simulink model "gap_generation_single_veh"  (R2019a)
settings: Solver=VariableStepAuto  StartTime=0.0  StopTime=35  FixedStep=0.1  MaxStep=0.05  RelTol=1e-3
libraries: simulink x21, powerlib_meascontrol x5, autolibshared x5
(part 2 of 3)

== system gap_generation_single_veh/Fo/Longitudinal Adjustments for Lane Change ==
  currentStates : Inport
  leaderStates : Inport  Port=2
  lcFlag : Inport  Port=3
  Enable : EnablePort
  Bus Selector : BusSelector  OutputSignals=X,Xdot,u
  Bus Selector1 : BusSelector  OutputSignals=X,Xdot
  Chart : Stateflow chart  BlockKeywords=__PRM__SERIALIZED__DATA__:Stateflow Chart,Stateflow Diagram  TreatAsAtomicUnit=on
  Gain3 : Gain  Gain=velFilterGain/10
  Headway error : Subsystem
  Input Saturation : Saturate  UpperLimit=maxComfAccel  LowerLimit=minComfAccel
  Integrator1 : Integrator  InitialCondition=vx0
  Mux : Mux  Inputs=2
  Rate Limiter : RateLimiter  RisingSlewLimit=maxComfJerk  FallingSlewLimit=minComfJerk  SampleTimeMode=inherited
  Saturation : Saturate  UpperLimit=maxAcceleration  LowerLimit=minAcceleration
  Scope3 : Scope  NumInputPorts=2
  Sum : Sum  Inputs=-+|
  Sum2 : Sum  Inputs=|+-
  Sum6 : Sum  Inputs=|+-
  Transport Delay : TransportDelay  DelayTime=0.01
  Transport Delay1 : TransportDelay  DelayTime=0.01
  Veh Following : Subsystem  TreatAsAtomicUnit=on
  Velocity Control : Subsystem  TreatAsAtomicUnit=on
  vMin : Constant  Value=vMin
  u : Outport  InitialOutput=0
  errors : Outport  Port=2  OutputWhenDisabled=reset  InitialOutput=[0, 0]
  gap : Outport  Port=3  OutputWhenDisabled=reset  InitialOutput=[0]
  wires:
  Transport Delay1/1 -> Velocity Control/1(intReset)
  Chart/1(state) -> Transport Delay1/1
  Transport Delay/1 -> Scope3/1, Input Saturation/1
  Velocity Control/1(Out1) -> Chart/2(uVelControl)  "uVelControl"
  Veh Following/1(u) -> Chart/3(uVehFoll)  "uVehFoll"
  Saturation/1 -> Integrator1/1
  Input Saturation/1 -> Rate Limiter/1
  Rate Limiter/1 -> Scope3/2, u/1  "sat(u)"
  Headway error/1(eh) -> Veh Following/1(eh), Mux/1  "eh"
  Sum2/1 -> Gain3/1
  Sum6/1 -> Velocity Control/2(ev), Chart/1(velDiff)
  Bus Selector1/2 -> Sum2/1  "<Xdot>"
  Chart/2(u) -> Transport Delay/1  "u"
  Sum/1 -> Veh Following/2(ev), Mux/2  "ev"
  vMin/1 -> Sum6/1
  Gain3/1 -> Saturation/1
  Integrator1/1 -> Sum2/2, Sum/2
  Mux/1 -> errors/1
  Bus Selector/2 -> Sum6/2, Sum/1, Headway error/2(vf)  "<Xdot>"
  Bus Selector/1 -> Headway error/1(xf)  "<X>"
  currentStates/1 -> Bus Selector/1
  Headway error/2("gap ") -> gap/1
  leaderStates/1 -> Bus Selector1/1
  Bus Selector1/1 -> Headway error/3(xl)  "<X>"
  lcFlag/1 -> Headway error/4(lcFlag)
  Bus Selector/3 -> Veh Following/3(realInput)  "<u>"

== system gap_generation_single_veh/Fo/Regular Vehicle Following ==
  currentStates : Inport
  leaderStates : Inport  Port=2
  lcFlag : Inport  Port=3
  AND1 : Logic  IconShape=distinctive  AllPortsSameDT=off  OutDataTypeStr=boolean
  Bus Selector : BusSelector  OutputSignals=X,Xdot,u
  Bus Selector1 : BusSelector  OutputSignals=X,Xdot
  Compare To Constant : simulink/Logic and Bit Operations/Compare To Constant  relop=<  const=2*maxHeadwayError  OutDataTypeStr=boolean
  Gain3 : Gain  Gain=velFilterGain
  Headway error : Subsystem
  Integrator1 : Integrator  InitialCondition=vx0
  Merge : Merge
  Mux : Mux  Inputs=2
  NOT : Logic  Operator=NOT  IconShape=distinctive  AllPortsSameDT=off  OutDataTypeStr=boolean
  NOT1 : Logic  Operator=NOT  IconShape=distinctive  AllPortsSameDT=off  OutDataTypeStr=boolean
  Rate Limiter : RateLimiter  RisingSlewLimit=maxJerk  FallingSlewLimit=minJerk  SampleTimeMode=inherited
  Rate Limiter1 : RateLimiter  RisingSlewLimit=maxComfJerk  FallingSlewLimit=minComfJerk  SampleTimeMode=inherited
  Saturation : Saturate  UpperLimit=maxAcceleration  LowerLimit=minAcceleration
  Sum : Sum  Inputs=-+|
  Sum2 : Sum  Inputs=|+-
  Switch1 : Switch  Criteria=u2 > Threshold
  Transport Delay : TransportDelay  DelayTime=0.01
  Veh Following : Subsystem  TreatAsAtomicUnit=on
  Velocity Control : Subsystem  TreatAsAtomicUnit=on
  comf saturation : Saturate  UpperLimit=maxComfAccel  LowerLimit=minComfAccel
  safe saturation : Saturate  UpperLimit=maxAcceleration  LowerLimit=minAcceleration
  u : Outport
  errors : Outport  Port=2
  gap : Outport  Port=3
  wires:
  NOT1/1 -> Velocity Control/Enable
  lcFlag/1 -> Headway error/4(lcFlag), AND1/1
  NOT/1 -> AND1/2
  Bus Selector/3 -> Veh Following/3(realInput)  "<u>"
  Bus Selector1/1 -> Headway error/3(xl)  "<X>"
  Headway error/3(unsafeFlag) -> NOT/1
  Headway error/2("gap ") -> gap/1
  Headway error/1(eh) -> Compare To Constant/1, Veh Following/1(eh), Mux/1
  Mux/1 -> errors/1
  Transport Delay/1 -> comf saturation/1, safe saturation/1
  Merge/1 -> Transport Delay/1
  Velocity Control/1(Out1) -> Merge/2
  Compare To Constant/1 -> Veh Following/Enable, NOT1/1
  Veh Following/1(u) -> Merge/1
  Rate Limiter1/1 -> Switch1/1  "sat(u)"
  Switch1/1 -> u/1
  Rate Limiter/1 -> Switch1/3  "sat(u)"
  safe saturation/1 -> Rate Limiter/1
  AND1/1 -> Switch1/2
  comf saturation/1 -> Rate Limiter1/1
  leaderStates/1 -> Bus Selector1/1
  Bus Selector/1 -> Headway error/1(xf)  "<X>"
  currentStates/1 -> Bus Selector/1
  Sum/1 -> Velocity Control/1(ev), Veh Following/2(ev), Mux/2
  Sum2/1 -> Gain3/1
  Bus Selector1/2 -> Sum2/1  "<Xdot>"
  Integrator1/1 -> Sum/2, Sum2/2
  Saturation/1 -> Integrator1/1
  Gain3/1 -> Saturation/1
  Bus Selector/2 -> Headway error/2(vf), Sum/1  "<Xdot>"

== system gap_generation_single_veh/Ld/Longitudinal Adjustments for Lane Change ==
  currentStates : Inport
  leaderStates : Inport  Port=2
  lcFlag : Inport  Port=3
  Enable : EnablePort
  Bus Selector : BusSelector  OutputSignals=X,Xdot,u
  Bus Selector1 : BusSelector  OutputSignals=X,Xdot
  Chart : Stateflow chart  BlockKeywords=__PRM__SERIALIZED__DATA__:Stateflow Chart,Stateflow Diagram  TreatAsAtomicUnit=on
  Gain3 : Gain  Gain=velFilterGain/10
  Headway error : Subsystem
  Input Saturation : Saturate  UpperLimit=maxComfAccel  LowerLimit=minComfAccel
  Integrator1 : Integrator  InitialCondition=vx0
  Mux : Mux  Inputs=2
  Rate Limiter : RateLimiter  RisingSlewLimit=maxComfJerk  FallingSlewLimit=minComfJerk  SampleTimeMode=inherited
  Saturation : Saturate  UpperLimit=maxAcceleration  LowerLimit=minAcceleration
  Scope3 : Scope  NumInputPorts=2
  Sum : Sum  Inputs=-+|
  Sum2 : Sum  Inputs=|+-
  Sum6 : Sum  Inputs=|+-
  Transport Delay : TransportDelay  DelayTime=0.01
  Transport Delay1 : TransportDelay  DelayTime=0.01
  Veh Following : Subsystem  TreatAsAtomicUnit=on
  Velocity Control : Subsystem  TreatAsAtomicUnit=on
  vMin : Constant  Value=vMin
  u : Outport  InitialOutput=0
  errors : Outport  Port=2  OutputWhenDisabled=reset  InitialOutput=[0, 0]
  gap : Outport  Port=3  OutputWhenDisabled=reset  InitialOutput=[0]
  wires:
  Transport Delay1/1 -> Velocity Control/1(intReset)
  Chart/1(state) -> Transport Delay1/1
  Transport Delay/1 -> Scope3/1, Input Saturation/1
  Velocity Control/1(Out1) -> Chart/2(uVelControl)  "uVelControl"
  Veh Following/1(u) -> Chart/3(uVehFoll)  "uVehFoll"
  Saturation/1 -> Integrator1/1
  Input Saturation/1 -> Rate Limiter/1
  Rate Limiter/1 -> Scope3/2, u/1  "sat(u)"
  Headway error/1(eh) -> Veh Following/1(eh), Mux/1  "eh"
  Sum2/1 -> Gain3/1
  Sum6/1 -> Velocity Control/2(ev), Chart/1(velDiff)
  Bus Selector1/2 -> Sum2/1  "<Xdot>"
  Chart/2(u) -> Transport Delay/1  "u"
  Sum/1 -> Veh Following/2(ev), Mux/2  "ev"
  vMin/1 -> Sum6/1
  Gain3/1 -> Saturation/1
  Integrator1/1 -> Sum2/2, Sum/2
  Mux/1 -> errors/1
  Bus Selector/2 -> Sum6/2, Sum/1, Headway error/2(vf)  "<Xdot>"
  Bus Selector/1 -> Headway error/1(xf)  "<X>"
  currentStates/1 -> Bus Selector/1
  Headway error/2("gap ") -> gap/1
  leaderStates/1 -> Bus Selector1/1
  Bus Selector1/1 -> Headway error/3(xl)  "<X>"
  lcFlag/1 -> Headway error/4(lcFlag)
  Bus Selector/3 -> Veh Following/3(realInput)  "<u>"

== system gap_generation_single_veh/Ld/Regular Vehicle Following ==
  currentStates : Inport
  leaderStates : Inport  Port=2
  lcFlag : Inport  Port=3
  AND1 : Logic  IconShape=distinctive  AllPortsSameDT=off  OutDataTypeStr=boolean
  Bus Selector : BusSelector  OutputSignals=X,Xdot,u
  Bus Selector1 : BusSelector  OutputSignals=X,Xdot
  Compare To Constant : simulink/Logic and Bit Operations/Compare To Constant  relop=<  const=2*maxHeadwayError  OutDataTypeStr=boolean
  Gain3 : Gain  Gain=velFilterGain
  Headway error : Subsystem
  Integrator1 : Integrator  InitialCondition=vx0
  Merge : Merge
  Mux : Mux  Inputs=2
  NOT : Logic  Operator=NOT  IconShape=distinctive  AllPortsSameDT=off  OutDataTypeStr=boolean
  NOT1 : Logic  Operator=NOT  IconShape=distinctive  AllPortsSameDT=off  OutDataTypeStr=boolean
  Rate Limiter : RateLimiter  RisingSlewLimit=maxJerk  FallingSlewLimit=minJerk  SampleTimeMode=inherited
  Rate Limiter1 : RateLimiter  RisingSlewLimit=maxComfJerk  FallingSlewLimit=minComfJerk  SampleTimeMode=inherited
  Saturation : Saturate  UpperLimit=maxAcceleration  LowerLimit=minAcceleration
  Sum : Sum  Inputs=-+|
  Sum2 : Sum  Inputs=|+-
  Switch1 : Switch  Criteria=u2 > Threshold
  Transport Delay : TransportDelay  DelayTime=0.01
  Veh Following : Subsystem  TreatAsAtomicUnit=on
  Velocity Control : Subsystem  TreatAsAtomicUnit=on
  comf saturation : Saturate  UpperLimit=maxComfAccel  LowerLimit=minComfAccel
  safe saturation : Saturate  UpperLimit=maxAcceleration  LowerLimit=minAcceleration
  u : Outport
  errors : Outport  Port=2
  gap : Outport  Port=3
  wires:
  NOT1/1 -> Velocity Control/Enable
  lcFlag/1 -> Headway error/4(lcFlag), AND1/1
  NOT/1 -> AND1/2
  Bus Selector/3 -> Veh Following/3(realInput)  "<u>"
  Bus Selector1/1 -> Headway error/3(xl)  "<X>"
  Headway error/3(unsafeFlag) -> NOT/1
  Headway error/2("gap ") -> gap/1
  Headway error/1(eh) -> Compare To Constant/1, Veh Following/1(eh), Mux/1
  Mux/1 -> errors/1
  Transport Delay/1 -> comf saturation/1, safe saturation/1
  Merge/1 -> Transport Delay/1
  Velocity Control/1(Out1) -> Merge/2
  Compare To Constant/1 -> Veh Following/Enable, NOT1/1
  Veh Following/1(u) -> Merge/1
  Rate Limiter1/1 -> Switch1/1  "sat(u)"
  Switch1/1 -> u/1
  Rate Limiter/1 -> Switch1/3  "sat(u)"
  safe saturation/1 -> Rate Limiter/1
  AND1/1 -> Switch1/2
  comf saturation/1 -> Rate Limiter1/1
  leaderStates/1 -> Bus Selector1/1
  Bus Selector/1 -> Headway error/1(xf)  "<X>"
  currentStates/1 -> Bus Selector/1
  Sum/1 -> Velocity Control/1(ev), Veh Following/2(ev), Mux/2
  Sum2/1 -> Gain3/1
  Bus Selector1/2 -> Sum2/1  "<Xdot>"
  Integrator1/1 -> Sum/2, Sum2/2
  Saturation/1 -> Integrator1/1
  Gain3/1 -> Saturation/1
  Bus Selector/2 -> Headway error/2(vf), Sum/1  "<Xdot>"

== system gap_generation_single_veh/Lo/Longitudinal Adjustments for Lane Change ==
  currentStates : Inport
  leaderStates : Inport  Port=2
  lcFlag : Inport  Port=3
  Enable : EnablePort
  Bus Selector : BusSelector  OutputSignals=X,Xdot,u
  Bus Selector1 : BusSelector  OutputSignals=X,Xdot
  Chart : Stateflow chart  BlockKeywords=__PRM__SERIALIZED__DATA__:Stateflow Chart,Stateflow Diagram  TreatAsAtomicUnit=on
  Gain3 : Gain  Gain=velFilterGain/10
  Headway error : Subsystem
  Input Saturation : Saturate  UpperLimit=maxComfAccel  LowerLimit=minComfAccel
  Integrator1 : Integrator  InitialCondition=vx0
  Mux : Mux  Inputs=2
  Rate Limiter : RateLimiter  RisingSlewLimit=maxComfJerk  FallingSlewLimit=minComfJerk  SampleTimeMode=inherited
  Saturation : Saturate  UpperLimit=maxAcceleration  LowerLimit=minAcceleration
  Scope3 : Scope  NumInputPorts=2
  Sum : Sum  Inputs=-+|
  Sum2 : Sum  Inputs=|+-
  Sum6 : Sum  Inputs=|+-
  Transport Delay : TransportDelay  DelayTime=0.01
  Transport Delay1 : TransportDelay  DelayTime=0.01
  Veh Following : Subsystem  TreatAsAtomicUnit=on
  Velocity Control : Subsystem  TreatAsAtomicUnit=on
  vMin : Constant  Value=vMin
  u : Outport  InitialOutput=0
  errors : Outport  Port=2  OutputWhenDisabled=reset  InitialOutput=[0, 0]
  gap : Outport  Port=3  OutputWhenDisabled=reset  InitialOutput=[0]
  wires:
  Transport Delay1/1 -> Velocity Control/1(intReset)
  Chart/1(state) -> Transport Delay1/1
  Transport Delay/1 -> Scope3/1, Input Saturation/1
  Velocity Control/1(Out1) -> Chart/2(uVelControl)  "uVelControl"
  Veh Following/1(u) -> Chart/3(uVehFoll)  "uVehFoll"
  Saturation/1 -> Integrator1/1
  Input Saturation/1 -> Rate Limiter/1
  Rate Limiter/1 -> Scope3/2, u/1  "sat(u)"
  Headway error/1(eh) -> Veh Following/1(eh), Mux/1  "eh"
  Sum2/1 -> Gain3/1
  Sum6/1 -> Velocity Control/2(ev), Chart/1(velDiff)
  Bus Selector1/2 -> Sum2/1  "<Xdot>"
  Chart/2(u) -> Transport Delay/1  "u"
  Sum/1 -> Veh Following/2(ev), Mux/2  "ev"
  vMin/1 -> Sum6/1
  Gain3/1 -> Saturation/1
  Integrator1/1 -> Sum2/2, Sum/2
  Mux/1 -> errors/1
  Bus Selector/2 -> Sum6/2, Sum/1, Headway error/2(vf)  "<Xdot>"
  Bus Selector/1 -> Headway error/1(xf)  "<X>"
  currentStates/1 -> Bus Selector/1
  Headway error/2("gap ") -> gap/1
  leaderStates/1 -> Bus Selector1/1
  Bus Selector1/1 -> Headway error/3(xl)  "<X>"
  lcFlag/1 -> Headway error/4(lcFlag)
  Bus Selector/3 -> Veh Following/3(realInput)  "<u>"

== system gap_generation_single_veh/Lo/Regular Vehicle Following ==
  currentStates : Inport
  leaderStates : Inport  Port=2
  lcFlag : Inport  Port=3
  AND1 : Logic  IconShape=distinctive  AllPortsSameDT=off  OutDataTypeStr=boolean
  Bus Selector : BusSelector  OutputSignals=X,Xdot,u
  Bus Selector1 : BusSelector  OutputSignals=X,Xdot
  Compare To Constant : simulink/Logic and Bit Operations/Compare To Constant  relop=<  const=2*maxHeadwayError  OutDataTypeStr=boolean
  Gain3 : Gain  Gain=velFilterGain
  Headway error : Subsystem
  Integrator1 : Integrator  InitialCondition=vx0
  Merge : Merge
  Mux : Mux  Inputs=2
  NOT : Logic  Operator=NOT  IconShape=distinctive  AllPortsSameDT=off  OutDataTypeStr=boolean
  NOT1 : Logic  Operator=NOT  IconShape=distinctive  AllPortsSameDT=off  OutDataTypeStr=boolean
  Rate Limiter : RateLimiter  RisingSlewLimit=maxJerk  FallingSlewLimit=minJerk  SampleTimeMode=inherited
  Rate Limiter1 : RateLimiter  RisingSlewLimit=maxComfJerk  FallingSlewLimit=minComfJerk  SampleTimeMode=inherited
  Saturation : Saturate  UpperLimit=maxAcceleration  LowerLimit=minAcceleration
  Sum : Sum  Inputs=-+|
  Sum2 : Sum  Inputs=|+-
  Switch1 : Switch  Criteria=u2 > Threshold
  Transport Delay : TransportDelay  DelayTime=0.01
  Veh Following : Subsystem  TreatAsAtomicUnit=on
  Velocity Control : Subsystem  TreatAsAtomicUnit=on
  comf saturation : Saturate  UpperLimit=maxComfAccel  LowerLimit=minComfAccel
  safe saturation : Saturate  UpperLimit=maxAcceleration  LowerLimit=minAcceleration
  u : Outport
  errors : Outport  Port=2
  gap : Outport  Port=3
  wires:
  NOT1/1 -> Velocity Control/Enable
  lcFlag/1 -> Headway error/4(lcFlag), AND1/1
  NOT/1 -> AND1/2
  Bus Selector/3 -> Veh Following/3(realInput)  "<u>"
  Bus Selector1/1 -> Headway error/3(xl)  "<X>"
  Headway error/3(unsafeFlag) -> NOT/1
  Headway error/2("gap ") -> gap/1
  Headway error/1(eh) -> Compare To Constant/1, Veh Following/1(eh), Mux/1
  Mux/1 -> errors/1
  Transport Delay/1 -> comf saturation/1, safe saturation/1
  Merge/1 -> Transport Delay/1
  Velocity Control/1(Out1) -> Merge/2
  Compare To Constant/1 -> Veh Following/Enable, NOT1/1
  Veh Following/1(u) -> Merge/1
  Rate Limiter1/1 -> Switch1/1  "sat(u)"
  Switch1/1 -> u/1
  Rate Limiter/1 -> Switch1/3  "sat(u)"
  safe saturation/1 -> Rate Limiter/1
  AND1/1 -> Switch1/2
  comf saturation/1 -> Rate Limiter1/1
  leaderStates/1 -> Bus Selector1/1
  Bus Selector/1 -> Headway error/1(xf)  "<X>"
  currentStates/1 -> Bus Selector/1
  Sum/1 -> Velocity Control/1(ev), Veh Following/2(ev), Mux/2
  Sum2/1 -> Gain3/1
  Bus Selector1/2 -> Sum2/1  "<Xdot>"
  Integrator1/1 -> Sum/2, Sum2/2
  Saturation/1 -> Integrator1/1
  Gain3/1 -> Saturation/1
  Bus Selector/2 -> Headway error/2(vf), Sum/1  "<Xdot>"

== system gap_generation_single_veh/p1/Longitudinal Adjustments for Lane Change ==
  currentStates : Inport
  leaderStates : Inport  Port=2
  lcFlag : Inport  Port=3
  Enable : EnablePort
  Bus Selector : BusSelector  OutputSignals=X,Xdot,u
  Bus Selector1 : BusSelector  OutputSignals=X,Xdot
  Chart : Stateflow chart  BlockKeywords=__PRM__SERIALIZED__DATA__:Stateflow Chart,Stateflow Diagram  TreatAsAtomicUnit=on
  Gain3 : Gain  Gain=velFilterGain/10
  Headway error : Subsystem
  Input Saturation : Saturate  UpperLimit=maxComfAccel  LowerLimit=minComfAccel
  Integrator1 : Integrator  InitialCondition=vx0
  Mux : Mux  Inputs=2
  Rate Limiter : RateLimiter  RisingSlewLimit=maxComfJerk  FallingSlewLimit=minComfJerk  SampleTimeMode=inherited
  Saturation : Saturate  UpperLimit=maxAcceleration  LowerLimit=minAcceleration
  Scope3 : Scope  NumInputPorts=2
  Sum : Sum  Inputs=-+|
  Sum2 : Sum  Inputs=|+-
  Sum6 : Sum  Inputs=|+-
  Transport Delay : TransportDelay  DelayTime=0.01
  Transport Delay1 : TransportDelay  DelayTime=0.01
  Veh Following : Subsystem  TreatAsAtomicUnit=on
  Velocity Control : Subsystem  TreatAsAtomicUnit=on
  vMin : Constant  Value=vMin
  u : Outport  InitialOutput=0
  errors : Outport  Port=2  OutputWhenDisabled=reset  InitialOutput=[0, 0]
  gap : Outport  Port=3  OutputWhenDisabled=reset  InitialOutput=[0]
  wires:
  Transport Delay1/1 -> Velocity Control/1(intReset)
  Chart/1(state) -> Transport Delay1/1
  Transport Delay/1 -> Scope3/1, Input Saturation/1
  Velocity Control/1(Out1) -> Chart/2(uVelControl)  "uVelControl"
  Veh Following/1(u) -> Chart/3(uVehFoll)  "uVehFoll"
  Saturation/1 -> Integrator1/1
  Input Saturation/1 -> Rate Limiter/1
  Rate Limiter/1 -> Scope3/2, u/1  "sat(u)"
  Headway error/1(eh) -> Veh Following/1(eh), Mux/1  "eh"
  Sum2/1 -> Gain3/1
  Sum6/1 -> Velocity Control/2(ev), Chart/1(velDiff)
  Bus Selector1/2 -> Sum2/1  "<Xdot>"
  Chart/2(u) -> Transport Delay/1  "u"
  Sum/1 -> Veh Following/2(ev), Mux/2  "ev"
  vMin/1 -> Sum6/1
  Gain3/1 -> Saturation/1
  Integrator1/1 -> Sum2/2, Sum/2
  Mux/1 -> errors/1
  Bus Selector/2 -> Sum6/2, Sum/1, Headway error/2(vf)  "<Xdot>"
  Bus Selector/1 -> Headway error/1(xf)  "<X>"
  currentStates/1 -> Bus Selector/1
  Headway error/2("gap ") -> gap/1
  leaderStates/1 -> Bus Selector1/1
  Bus Selector1/1 -> Headway error/3(xl)  "<X>"
  lcFlag/1 -> Headway error/4(lcFlag)
  Bus Selector/3 -> Veh Following/3(realInput)  "<u>"

== system gap_generation_single_veh/p1/Regular Vehicle Following ==
  currentStates : Inport
  leaderStates : Inport  Port=2
  lcFlag : Inport  Port=3
  AND1 : Logic  IconShape=distinctive  AllPortsSameDT=off  OutDataTypeStr=boolean
  Bus Selector : BusSelector  OutputSignals=X,Xdot,u
  Bus Selector1 : BusSelector  OutputSignals=X,Xdot
  Compare To Constant : simulink/Logic and Bit Operations/Compare To Constant  relop=<  const=2*maxHeadwayError  OutDataTypeStr=boolean
  Gain3 : Gain  Gain=velFilterGain
  Headway error : Subsystem
  Integrator1 : Integrator  InitialCondition=vx0
  Merge : Merge
  Mux : Mux  Inputs=2
  NOT : Logic  Operator=NOT  IconShape=distinctive  AllPortsSameDT=off  OutDataTypeStr=boolean
  NOT1 : Logic  Operator=NOT  IconShape=distinctive  AllPortsSameDT=off  OutDataTypeStr=boolean
  Rate Limiter : RateLimiter  RisingSlewLimit=maxJerk  FallingSlewLimit=minJerk  SampleTimeMode=inherited
  Rate Limiter1 : RateLimiter  RisingSlewLimit=maxComfJerk  FallingSlewLimit=minComfJerk  SampleTimeMode=inherited
  Saturation : Saturate  UpperLimit=maxAcceleration  LowerLimit=minAcceleration
  Sum : Sum  Inputs=-+|
  Sum2 : Sum  Inputs=|+-
  Switch1 : Switch  Criteria=u2 > Threshold
  Transport Delay : TransportDelay  DelayTime=0.01
  Veh Following : Subsystem  TreatAsAtomicUnit=on
  Velocity Control : Subsystem  TreatAsAtomicUnit=on
  comf saturation : Saturate  UpperLimit=maxComfAccel  LowerLimit=minComfAccel
  safe saturation : Saturate  UpperLimit=maxAcceleration  LowerLimit=minAcceleration
  u : Outport
  errors : Outport  Port=2
  gap : Outport  Port=3
  wires:
  NOT1/1 -> Velocity Control/Enable
  lcFlag/1 -> Headway error/4(lcFlag), AND1/1
  NOT/1 -> AND1/2
  Bus Selector/3 -> Veh Following/3(realInput)  "<u>"
  Bus Selector1/1 -> Headway error/3(xl)  "<X>"
  Headway error/3(unsafeFlag) -> NOT/1
  Headway error/2("gap ") -> gap/1
  Headway error/1(eh) -> Compare To Constant/1, Veh Following/1(eh), Mux/1
  Mux/1 -> errors/1
  Transport Delay/1 -> comf saturation/1, safe saturation/1
  Merge/1 -> Transport Delay/1
  Velocity Control/1(Out1) -> Merge/2
  Compare To Constant/1 -> Veh Following/Enable, NOT1/1
  Veh Following/1(u) -> Merge/1
  Rate Limiter1/1 -> Switch1/1  "sat(u)"
  Switch1/1 -> u/1
  Rate Limiter/1 -> Switch1/3  "sat(u)"
  safe saturation/1 -> Rate Limiter/1
  AND1/1 -> Switch1/2
  comf saturation/1 -> Rate Limiter1/1
  leaderStates/1 -> Bus Selector1/1
  Bus Selector/1 -> Headway error/1(xf)  "<X>"
  currentStates/1 -> Bus Selector/1
  Sum/1 -> Velocity Control/1(ev), Veh Following/2(ev), Mux/2
  Sum2/1 -> Gain3/1
  Bus Selector1/2 -> Sum2/1  "<Xdot>"
  Integrator1/1 -> Sum/2, Sum2/2
  Saturation/1 -> Integrator1/1
  Gain3/1 -> Saturation/1
  Bus Selector/2 -> Headway error/2(vf), Sum/1  "<Xdot>"

== system gap_generation_single_veh/Fd/Longitudinal Adjustments for Lane Change/Headway error ==
  xf : Inport
  vf : Inport  Port=2
  xl : Inport  Port=3
  lcFlag : Inport  Port=4
  Demux : Demux  Outputs=2
  Integrator : Integrator  InitialCondition=h
  Multiply : Product
  Mux : Mux  Inputs=2
  Mux1 : Mux  Inputs=2
  Sum : Sum  Inputs=-+|
  Sum1 : Sum  Inputs=++|
  Sum2 : Sum  Inputs=+-|
  Sum3 : Sum  Inputs=|++
  Sum4 : Sum  Inputs=|+-
  Switch : Switch  Criteria=u2 > Threshold
  d0 : Constant  Value=d0
  d0Lc : Constant  Value=d0Lc
  h : Constant  Value=h
  hFilterGain : Gain  Gain=hFilterGain
  hLc : Constant  Value=hLc
  vLen : Constant  Value=lr+lf
  eh : Outport
  "gap " : Outport  Port=2
  wires:
  vLen/1 -> Sum1/1
  Multiply/1 -> Sum3/1
  Sum/1 -> "gap "/1, Sum2/1  "gap"
  xf/1 -> Sum1/2
  Sum3/1 -> Sum2/2  "desired  gap"
  vf/1 -> Multiply/1
  Sum1/1 -> Sum/1  "x (front bumber)"
  xl/1 -> Sum/2
  h/1 -> Mux/1
  Switch/1 -> Sum4/1
  hFilterGain/1 -> Integrator/1
  Sum4/1 -> hFilterGain/1
  Integrator/1 -> Sum4/2, Demux/1
  lcFlag/1 -> Switch/2
  Sum2/1 -> eh/1
  d0/1 -> Mux/2
  Mux/1 -> Switch/3
  hLc/1 -> Mux1/1
  d0Lc/1 -> Mux1/2
  Mux1/1 -> Switch/1
  Demux/1 -> Multiply/2  "time headway"
  Demux/2 -> Sum3/2  "gap at  standstill"

== system gap_generation_single_veh/Fd/Longitudinal Adjustments for Lane Change/Veh Following ==
  eh : Inport
  ev : Inport  Port=2
  realInput : Inport  Port=3
  Anti-windup gain : Gain  Gain=sqrt(Ki/Kd)
  Integrator : Integrator
  Kd : Gain  Gain=Kd
  Ki : Gain  Gain=Ki
  Kp : Gain  Gain=Kp
  Saturation1 : Saturate  UpperLimit=maxHeadwayError  LowerLimit=minHeadwayError
  Scope : Scope  NumInputPorts=3
  Sum : Sum  Inputs=|-+
  Sum1 : Sum  Inputs=+++
  Sum5 : Sum  Inputs=-+|
  u : Outport
  wires:
  ev/1 -> Kd/1
  Ki/1 -> Sum5/2
  Anti-windup gain/1 -> Sum5/1
  Sum5/1 -> Integrator/1
  Integrator/1 -> Scope/1, Sum1/1
  Kp/1 -> Scope/2, Sum1/2
  Kd/1 -> Scope/3, Sum1/3
  Saturation1/1 -> Kp/1, Ki/1
  eh/1 -> Saturation1/1
  Sum1/1 -> Sum/2, u/1
  realInput/1 -> Sum/1
  Sum/1 -> Anti-windup gain/1

== system gap_generation_single_veh/Fd/Longitudinal Adjustments for Lane Change/Velocity Control ==
  note: Velocity control
  intReset : Inport
  ev : Inport  Port=2
  Integrator2 : Integrator  ExternalReset=rising
  Sum3 : Sum
  velKi : Gain  Gain=velKi
  velKp : Gain  Gain=velKp
  Out1 : Outport
  wires:
  Integrator2/1 -> velKi/1
  velKi/1 -> Sum3/2
  Sum3/1 -> Out1/1
  velKp/1 -> Sum3/1
  ev/1 -> velKp/1, Integrator2/1
  intReset/1 -> Integrator2/2

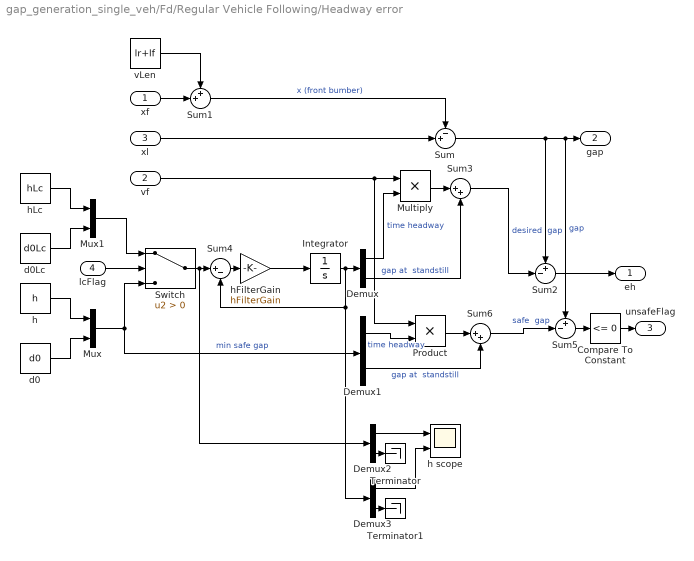
== system gap_generation_single_veh/Fd/Regular Vehicle Following/Headway error ==
  xf : Inport
  vf : Inport  Port=2
  xl : Inport  Port=3
  lcFlag : Inport  Port=4
  Compare To Constant : simulink/Logic and Bit Operations/Compare To Constant  relop=<=  const=0  OutDataTypeStr=boolean
  Demux{,1..3} (4 alike) : Demux  Outputs=2
  Integrator : Integrator  InitialCondition=[h d0]
  Multiply : Product
  Mux : Mux  Inputs=2
  Mux1 : Mux  Inputs=2
  Product : Product
  Sum : Sum  Inputs=-+|
  Sum1 : Sum  Inputs=++|
  Sum2 : Sum  Inputs=+-|
  Sum3 : Sum  Inputs=|++
  Sum4 : Sum  Inputs=|+-
  Sum5 : Sum  Inputs=+-|
  Sum6 : Sum  Inputs=|++
  Switch : Switch  Criteria=u2 > Threshold
  Terminator : Terminator
  Terminator1 : Terminator
  d0 : Constant  Value=d0
  d0Lc : Constant  Value=d0Lc
  h : Constant  Value=h
  h scope : Scope  NumInputPorts=2
  hFilterGain : Gain  Gain=hFilterGain
  hLc : Constant  Value=hLc
  vLen : Constant  Value=lr+lf
  eh : Outport
  "gap " : Outport  Port=2
  unsafeFlag : Outport  Port=3
  wires:
  vLen/1 -> Sum1/1
  Multiply/1 -> Sum3/1
  Sum/1 -> Sum5/1, "gap "/1, Sum2/1  "gap"
  xf/1 -> Sum1/2
  Sum3/1 -> Sum2/2  "desired  gap"
  vf/1 -> Product/1, Multiply/1
  Sum1/1 -> Sum/1  "x (front bumber)"
  xl/1 -> Sum/2
  h/1 -> Mux/1
  Switch/1 -> Demux2/1, Sum4/1
  Sum4/1 -> hFilterGain/1
  Integrator/1 -> Demux3/1, Sum4/2, Demux/1
  lcFlag/1 -> Switch/2
  Sum2/1 -> eh/1
  d0/1 -> Mux/2
  Mux/1 -> Demux1/1, Switch/3  "min safe gap"
  hLc/1 -> Mux1/1
  d0Lc/1 -> Mux1/2
  Mux1/1 -> Switch/1
  Demux/1 -> Multiply/2  "time headway"
  Demux/2 -> Sum3/2  "gap at  standstill"
  hFilterGain/1 -> Integrator/1
  Sum5/1 -> Compare To Constant/1
  Compare To Constant/1 -> unsafeFlag/1
  Demux1/1 -> Product/2  "time headway"
  Product/1 -> Sum6/1
  Demux1/2 -> Sum6/2  "gap at  standstill"
  Sum6/1 -> Sum5/2  "safe  gap"
  Demux2/1 -> h scope/1
  Demux3/1 -> h scope/2
  Demux2/2 -> Terminator/1
  Demux3/2 -> Terminator1/1

== system gap_generation_single_veh/Fd/Regular Vehicle Following/Veh Following ==
  eh : Inport
  ev : Inport  Port=2
  realInput : Inport  Port=3
  Enable : EnablePort
  Anti-windup gain : Gain  Gain=sqrt(Ki/Kd)
  Integrator : Integrator
  Kd : Gain  Gain=Kd
  Ki : Gain  Gain=Ki
  Kp : Gain  Gain=Kp
  Saturation1 : Saturate  UpperLimit=maxHeadwayError  LowerLimit=minHeadwayError
  Scope : Scope  NumInputPorts=3
  Sum : Sum  Inputs=|-+
  Sum1 : Sum  Inputs=+++
  Sum5 : Sum  Inputs=-+|
  u : Outport
  wires:
  ev/1 -> Kd/1
  Ki/1 -> Sum5/2
  Anti-windup gain/1 -> Sum5/1
  Sum5/1 -> Integrator/1
  Integrator/1 -> Scope/1, Sum1/1
  Kp/1 -> Scope/2, Sum1/2
  Kd/1 -> Scope/3, Sum1/3
  Saturation1/1 -> Kp/1, Ki/1
  eh/1 -> Saturation1/1
  Sum1/1 -> Sum/2, u/1
  realInput/1 -> Sum/1
  Sum/1 -> Anti-windup gain/1

== system gap_generation_single_veh/Fd/Regular Vehicle Following/Velocity Control ==
  note: Velocity control
  ev : Inport
  Enable : EnablePort
  Integrator2 : Integrator
  Sum3 : Sum
  velKi : Gain  Gain=velKi
  velKp : Gain  Gain=velKp
  Out1 : Outport
  wires:
  Integrator2/1 -> velKi/1
  velKi/1 -> Sum3/2
  Sum3/1 -> Out1/1
  velKp/1 -> Sum3/1
  ev/1 -> velKp/1, Integrator2/1

== system gap_generation_single_veh/Fo/Longitudinal Adjustments for Lane Change/Headway error ==
  xf : Inport
  vf : Inport  Port=2
  xl : Inport  Port=3
  lcFlag : Inport  Port=4
  Demux : Demux  Outputs=2
  Integrator : Integrator  InitialCondition=h
  Multiply : Product
  Mux : Mux  Inputs=2
  Mux1 : Mux  Inputs=2
  Sum : Sum  Inputs=-+|
  Sum1 : Sum  Inputs=++|
  Sum2 : Sum  Inputs=+-|
  Sum3 : Sum  Inputs=|++
  Sum4 : Sum  Inputs=|+-
  Switch : Switch  Criteria=u2 > Threshold
  d0 : Constant  Value=d0
  d0Lc : Constant  Value=d0Lc
  h : Constant  Value=h
  hFilterGain : Gain  Gain=hFilterGain
  hLc : Constant  Value=hLc
  vLen : Constant  Value=lr+lf
  eh : Outport
  "gap " : Outport  Port=2
  wires:
  Demux/2 -> Sum3/2  "gap at  standstill"
  Demux/1 -> Multiply/2  "time headway"
  Mux1/1 -> Switch/1
  d0Lc/1 -> Mux1/2
  hLc/1 -> Mux1/1
  Mux/1 -> Switch/3
  d0/1 -> Mux/2
  Sum2/1 -> eh/1
  lcFlag/1 -> Switch/2
  Integrator/1 -> Demux/1, Sum4/2
  Sum4/1 -> hFilterGain/1
  hFilterGain/1 -> Integrator/1
  Switch/1 -> Sum4/1
  h/1 -> Mux/1
  xl/1 -> Sum/2
  Sum1/1 -> Sum/1  "x (front bumber)"
  vf/1 -> Multiply/1
  Sum3/1 -> Sum2/2  "desired  gap"
  xf/1 -> Sum1/2
  Sum/1 -> Sum2/1, "gap "/1  "gap"
  Multiply/1 -> Sum3/1
  vLen/1 -> Sum1/1

== system gap_generation_single_veh/Fo/Longitudinal Adjustments for Lane Change/Veh Following ==
  eh : Inport
  ev : Inport  Port=2
  realInput : Inport  Port=3
  Anti-windup gain : Gain  Gain=sqrt(Ki/Kd)
  Integrator : Integrator
  Kd : Gain  Gain=Kd
  Ki : Gain  Gain=Ki
  Kp : Gain  Gain=Kp
  Saturation1 : Saturate  UpperLimit=maxHeadwayError  LowerLimit=minHeadwayError
  Scope : Scope  NumInputPorts=3
  Sum : Sum  Inputs=|-+
  Sum1 : Sum  Inputs=+++
  Sum5 : Sum  Inputs=-+|
  u : Outport
  wires:
  Sum/1 -> Anti-windup gain/1
  realInput/1 -> Sum/1
  Sum1/1 -> u/1, Sum/2
  eh/1 -> Saturation1/1
  Saturation1/1 -> Ki/1, Kp/1
  Kd/1 -> Sum1/3, Scope/3
  Kp/1 -> Sum1/2, Scope/2
  Integrator/1 -> Sum1/1, Scope/1
  Sum5/1 -> Integrator/1
  Anti-windup gain/1 -> Sum5/1
  Ki/1 -> Sum5/2
  ev/1 -> Kd/1

== system gap_generation_single_veh/Fo/Longitudinal Adjustments for Lane Change/Velocity Control ==
  note: Velocity control
  intReset : Inport
  ev : Inport  Port=2
  Integrator2 : Integrator  ExternalReset=rising
  Sum3 : Sum
  velKi : Gain  Gain=velKi
  velKp : Gain  Gain=velKp
  Out1 : Outport
  wires:
  intReset/1 -> Integrator2/2
  ev/1 -> Integrator2/1, velKp/1
  velKp/1 -> Sum3/1
  Sum3/1 -> Out1/1
  velKi/1 -> Sum3/2
  Integrator2/1 -> velKi/1

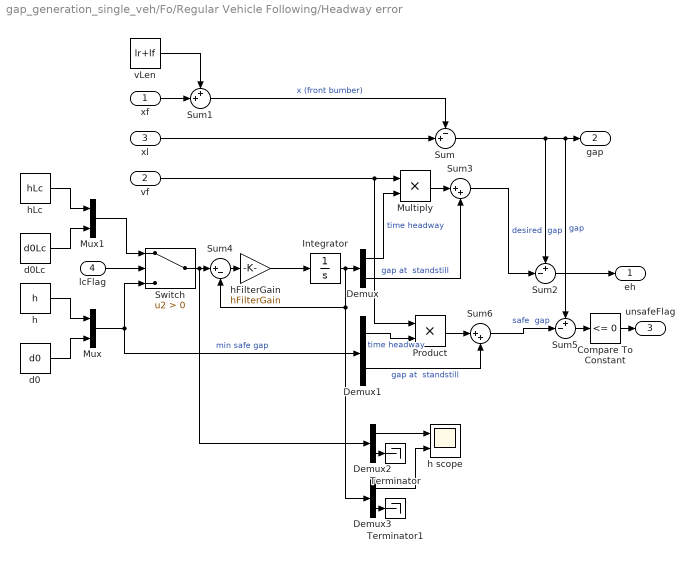
== system gap_generation_single_veh/Fo/Regular Vehicle Following/Headway error ==
  xf : Inport
  vf : Inport  Port=2
  xl : Inport  Port=3
  lcFlag : Inport  Port=4
  Compare To Constant : simulink/Logic and Bit Operations/Compare To Constant  relop=<=  const=0  OutDataTypeStr=boolean
  Demux{,1..3} (4 alike) : Demux  Outputs=2
  Integrator : Integrator  InitialCondition=[h d0]
  Multiply : Product
  Mux : Mux  Inputs=2
  Mux1 : Mux  Inputs=2
  Product : Product
  Sum : Sum  Inputs=-+|
  Sum1 : Sum  Inputs=++|
  Sum2 : Sum  Inputs=+-|
  Sum3 : Sum  Inputs=|++
  Sum4 : Sum  Inputs=|+-
  Sum5 : Sum  Inputs=+-|
  Sum6 : Sum  Inputs=|++
  Switch : Switch  Criteria=u2 > Threshold
  Terminator : Terminator
  Terminator1 : Terminator
  d0 : Constant  Value=d0
  d0Lc : Constant  Value=d0Lc
  h : Constant  Value=h
  h scope : Scope  NumInputPorts=2
  hFilterGain : Gain  Gain=hFilterGain
  hLc : Constant  Value=hLc
  vLen : Constant  Value=lr+lf
  eh : Outport
  "gap " : Outport  Port=2
  unsafeFlag : Outport  Port=3
  wires:
  Demux3/2 -> Terminator1/1
  Demux2/2 -> Terminator/1
  Demux3/1 -> h scope/2
  Demux2/1 -> h scope/1
  Sum6/1 -> Sum5/2  "safe  gap"
  Demux1/2 -> Sum6/2  "gap at  standstill"
  Product/1 -> Sum6/1
  Demux1/1 -> Product/2  "time headway"
  Compare To Constant/1 -> unsafeFlag/1
  Sum5/1 -> Compare To Constant/1
  hFilterGain/1 -> Integrator/1
  Demux/2 -> Sum3/2  "gap at  standstill"
  Demux/1 -> Multiply/2  "time headway"
  Mux1/1 -> Switch/1
  d0Lc/1 -> Mux1/2
  hLc/1 -> Mux1/1
  Mux/1 -> Switch/3, Demux1/1  "min safe gap"
  d0/1 -> Mux/2
  Sum2/1 -> eh/1
  lcFlag/1 -> Switch/2
  Integrator/1 -> Demux/1, Sum4/2, Demux3/1
  Sum4/1 -> hFilterGain/1
  Switch/1 -> Sum4/1, Demux2/1
  h/1 -> Mux/1
  xl/1 -> Sum/2
  Sum1/1 -> Sum/1  "x (front bumber)"
  vf/1 -> Multiply/1, Product/1
  Sum3/1 -> Sum2/2  "desired  gap"
  xf/1 -> Sum1/2
  Sum/1 -> Sum2/1, "gap "/1, Sum5/1  "gap"
  Multiply/1 -> Sum3/1
  vLen/1 -> Sum1/1

== system gap_generation_single_veh/Fo/Regular Vehicle Following/Veh Following ==
  eh : Inport
  ev : Inport  Port=2
  realInput : Inport  Port=3
  Enable : EnablePort
  Anti-windup gain : Gain  Gain=sqrt(Ki/Kd)
  Integrator : Integrator
  Kd : Gain  Gain=Kd
  Ki : Gain  Gain=Ki
  Kp : Gain  Gain=Kp
  Saturation1 : Saturate  UpperLimit=maxHeadwayError  LowerLimit=minHeadwayError
  Scope : Scope  NumInputPorts=3
  Sum : Sum  Inputs=|-+
  Sum1 : Sum  Inputs=+++
  Sum5 : Sum  Inputs=-+|
  u : Outport
  wires:
  Sum/1 -> Anti-windup gain/1
  realInput/1 -> Sum/1
  Sum1/1 -> u/1, Sum/2
  eh/1 -> Saturation1/1
  Saturation1/1 -> Ki/1, Kp/1
  Kd/1 -> Sum1/3, Scope/3
  Kp/1 -> Sum1/2, Scope/2
  Integrator/1 -> Sum1/1, Scope/1
  Sum5/1 -> Integrator/1
  Anti-windup gain/1 -> Sum5/1
  Ki/1 -> Sum5/2
  ev/1 -> Kd/1

== system gap_generation_single_veh/Fo/Regular Vehicle Following/Velocity Control ==
  note: Velocity control
  ev : Inport
  Enable : EnablePort
  Integrator2 : Integrator
  Sum3 : Sum
  velKi : Gain  Gain=velKi
  velKp : Gain  Gain=velKp
  Out1 : Outport
  wires:
  ev/1 -> Integrator2/1, velKp/1
  velKp/1 -> Sum3/1
  Sum3/1 -> Out1/1
  velKi/1 -> Sum3/2
  Integrator2/1 -> velKi/1

== system gap_generation_single_veh/Ld/Longitudinal Adjustments for Lane Change/Headway error ==
  xf : Inport
  vf : Inport  Port=2
  xl : Inport  Port=3
  lcFlag : Inport  Port=4
  Demux : Demux  Outputs=2
  Integrator : Integrator  InitialCondition=h
  Multiply : Product
  Mux : Mux  Inputs=2
  Mux1 : Mux  Inputs=2
  Sum : Sum  Inputs=-+|
  Sum1 : Sum  Inputs=++|
  Sum2 : Sum  Inputs=+-|
  Sum3 : Sum  Inputs=|++
  Sum4 : Sum  Inputs=|+-
  Switch : Switch  Criteria=u2 > Threshold
  d0 : Constant  Value=d0
  d0Lc : Constant  Value=d0Lc
  h : Constant  Value=h
  hFilterGain : Gain  Gain=hFilterGain
  hLc : Constant  Value=hLc
  vLen : Constant  Value=lr+lf
  eh : Outport
  "gap " : Outport  Port=2
  wires:
  Demux/2 -> Sum3/2  "gap at  standstill"
  Demux/1 -> Multiply/2  "time headway"
  Mux1/1 -> Switch/1
  d0Lc/1 -> Mux1/2
  hLc/1 -> Mux1/1
  Mux/1 -> Switch/3
  d0/1 -> Mux/2
  Sum2/1 -> eh/1
  lcFlag/1 -> Switch/2
  Integrator/1 -> Demux/1, Sum4/2
  Sum4/1 -> hFilterGain/1
  hFilterGain/1 -> Integrator/1
  Switch/1 -> Sum4/1
  h/1 -> Mux/1
  xl/1 -> Sum/2
  Sum1/1 -> Sum/1  "x (front bumber)"
  vf/1 -> Multiply/1
  Sum3/1 -> Sum2/2  "desired  gap"
  xf/1 -> Sum1/2
  Sum/1 -> Sum2/1, "gap "/1  "gap"
  Multiply/1 -> Sum3/1
  vLen/1 -> Sum1/1

== system gap_generation_single_veh/Ld/Longitudinal Adjustments for Lane Change/Veh Following ==
  eh : Inport
  ev : Inport  Port=2
  realInput : Inport  Port=3
  Anti-windup gain : Gain  Gain=sqrt(Ki/Kd)
  Integrator : Integrator
  Kd : Gain  Gain=Kd
  Ki : Gain  Gain=Ki
  Kp : Gain  Gain=Kp
  Saturation1 : Saturate  UpperLimit=maxHeadwayError  LowerLimit=minHeadwayError
  Scope : Scope  NumInputPorts=3
  Sum : Sum  Inputs=|-+
  Sum1 : Sum  Inputs=+++
  Sum5 : Sum  Inputs=-+|
  u : Outport
  wires:
  Sum/1 -> Anti-windup gain/1
  realInput/1 -> Sum/1
  Sum1/1 -> u/1, Sum/2
  eh/1 -> Saturation1/1
  Saturation1/1 -> Ki/1, Kp/1
  Kd/1 -> Sum1/3, Scope/3
  Kp/1 -> Sum1/2, Scope/2
  Integrator/1 -> Sum1/1, Scope/1
  Sum5/1 -> Integrator/1
  Anti-windup gain/1 -> Sum5/1
  Ki/1 -> Sum5/2
  ev/1 -> Kd/1

== system gap_generation_single_veh/Ld/Longitudinal Adjustments for Lane Change/Velocity Control ==
  note: Velocity control
  intReset : Inport
  ev : Inport  Port=2
  Integrator2 : Integrator  ExternalReset=rising
  Sum3 : Sum
  velKi : Gain  Gain=velKi
  velKp : Gain  Gain=velKp
  Out1 : Outport
  wires:
  intReset/1 -> Integrator2/2
  ev/1 -> Integrator2/1, velKp/1
  velKp/1 -> Sum3/1
  Sum3/1 -> Out1/1
  velKi/1 -> Sum3/2
  Integrator2/1 -> velKi/1

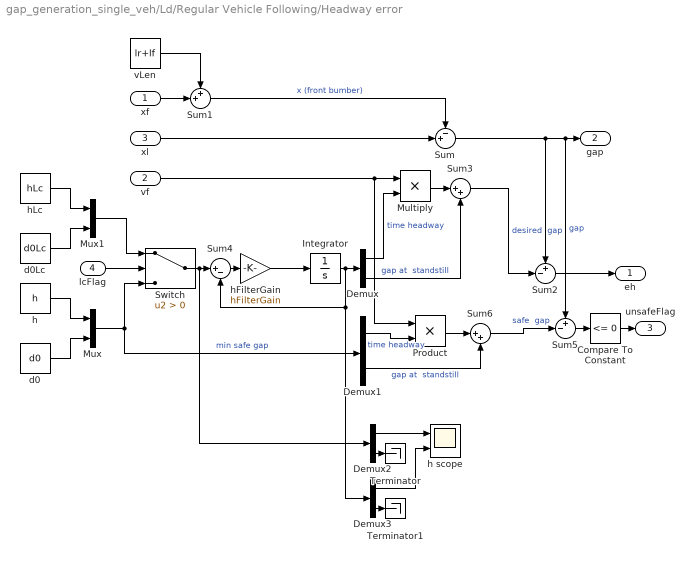
== system gap_generation_single_veh/Ld/Regular Vehicle Following/Headway error ==
  xf : Inport
  vf : Inport  Port=2
  xl : Inport  Port=3
  lcFlag : Inport  Port=4
  Compare To Constant : simulink/Logic and Bit Operations/Compare To Constant  relop=<=  const=0  OutDataTypeStr=boolean
  Demux{,1..3} (4 alike) : Demux  Outputs=2
  Integrator : Integrator  InitialCondition=[h d0]
  Multiply : Product
  Mux : Mux  Inputs=2
  Mux1 : Mux  Inputs=2
  Product : Product
  Sum : Sum  Inputs=-+|
  Sum1 : Sum  Inputs=++|
  Sum2 : Sum  Inputs=+-|
  Sum3 : Sum  Inputs=|++
  Sum4 : Sum  Inputs=|+-
  Sum5 : Sum  Inputs=+-|
  Sum6 : Sum  Inputs=|++
  Switch : Switch  Criteria=u2 > Threshold
  Terminator : Terminator
  Terminator1 : Terminator
  d0 : Constant  Value=d0
  d0Lc : Constant  Value=d0Lc
  h : Constant  Value=h
  h scope : Scope  NumInputPorts=2
  hFilterGain : Gain  Gain=hFilterGain
  hLc : Constant  Value=hLc
  vLen : Constant  Value=lr+lf
  eh : Outport
  "gap " : Outport  Port=2
  unsafeFlag : Outport  Port=3
  wires:
  Demux3/2 -> Terminator1/1
  Demux2/2 -> Terminator/1
  Demux3/1 -> h scope/2
  Demux2/1 -> h scope/1
  Sum6/1 -> Sum5/2  "safe  gap"
  Demux1/2 -> Sum6/2  "gap at  standstill"
  Product/1 -> Sum6/1
  Demux1/1 -> Product/2  "time headway"
  Compare To Constant/1 -> unsafeFlag/1
  Sum5/1 -> Compare To Constant/1
  hFilterGain/1 -> Integrator/1
  Demux/2 -> Sum3/2  "gap at  standstill"
  Demux/1 -> Multiply/2  "time headway"
  Mux1/1 -> Switch/1
  d0Lc/1 -> Mux1/2
  hLc/1 -> Mux1/1
  Mux/1 -> Switch/3, Demux1/1  "min safe gap"
  d0/1 -> Mux/2
  Sum2/1 -> eh/1
  lcFlag/1 -> Switch/2
  Integrator/1 -> Demux/1, Sum4/2, Demux3/1
  Sum4/1 -> hFilterGain/1
  Switch/1 -> Sum4/1, Demux2/1
  h/1 -> Mux/1
  xl/1 -> Sum/2
  Sum1/1 -> Sum/1  "x (front bumber)"
  vf/1 -> Multiply/1, Product/1
  Sum3/1 -> Sum2/2  "desired  gap"
  xf/1 -> Sum1/2
  Sum/1 -> Sum2/1, "gap "/1, Sum5/1  "gap"
  Multiply/1 -> Sum3/1
  vLen/1 -> Sum1/1

== system gap_generation_single_veh/Ld/Regular Vehicle Following/Veh Following ==
  eh : Inport
  ev : Inport  Port=2
  realInput : Inport  Port=3
  Enable : EnablePort
  Anti-windup gain : Gain  Gain=sqrt(Ki/Kd)
  Integrator : Integrator
  Kd : Gain  Gain=Kd
  Ki : Gain  Gain=Ki
  Kp : Gain  Gain=Kp
  Saturation1 : Saturate  UpperLimit=maxHeadwayError  LowerLimit=minHeadwayError
  Scope : Scope  NumInputPorts=3
  Sum : Sum  Inputs=|-+
  Sum1 : Sum  Inputs=+++
  Sum5 : Sum  Inputs=-+|
  u : Outport
  wires:
  Sum/1 -> Anti-windup gain/1
  realInput/1 -> Sum/1
  Sum1/1 -> u/1, Sum/2
  eh/1 -> Saturation1/1
  Saturation1/1 -> Ki/1, Kp/1
  Kd/1 -> Sum1/3, Scope/3
  Kp/1 -> Sum1/2, Scope/2
  Integrator/1 -> Sum1/1, Scope/1
  Sum5/1 -> Integrator/1
  Anti-windup gain/1 -> Sum5/1
  Ki/1 -> Sum5/2
  ev/1 -> Kd/1

== system gap_generation_single_veh/Ld/Regular Vehicle Following/Velocity Control ==
  note: Velocity control
  ev : Inport
  Enable : EnablePort
  Integrator2 : Integrator
  Sum3 : Sum
  velKi : Gain  Gain=velKi
  velKp : Gain  Gain=velKp
  Out1 : Outport
  wires:
  ev/1 -> Integrator2/1, velKp/1
  velKp/1 -> Sum3/1
  Sum3/1 -> Out1/1
  velKi/1 -> Sum3/2
  Integrator2/1 -> velKi/1

== system gap_generation_single_veh/Lo/Longitudinal Adjustments for Lane Change/Headway error ==
  xf : Inport
  vf : Inport  Port=2
  xl : Inport  Port=3
  lcFlag : Inport  Port=4
  Demux : Demux  Outputs=2
  Integrator : Integrator  InitialCondition=h
  Multiply : Product
  Mux : Mux  Inputs=2
  Mux1 : Mux  Inputs=2
  Sum : Sum  Inputs=-+|
  Sum1 : Sum  Inputs=++|
  Sum2 : Sum  Inputs=+-|
  Sum3 : Sum  Inputs=|++
  Sum4 : Sum  Inputs=|+-
  Switch : Switch  Criteria=u2 > Threshold
  d0 : Constant  Value=d0
  d0Lc : Constant  Value=d0Lc
  h : Constant  Value=h
  hFilterGain : Gain  Gain=hFilterGain
  hLc : Constant  Value=hLc
  vLen : Constant  Value=lr+lf
  eh : Outport
  "gap " : Outport  Port=2
  wires:
  Demux/2 -> Sum3/2  "gap at  standstill"
  Demux/1 -> Multiply/2  "time headway"
  Mux1/1 -> Switch/1
  d0Lc/1 -> Mux1/2
  hLc/1 -> Mux1/1
  Mux/1 -> Switch/3
  d0/1 -> Mux/2
  Sum2/1 -> eh/1
  lcFlag/1 -> Switch/2
  Integrator/1 -> Demux/1, Sum4/2
  Sum4/1 -> hFilterGain/1
  hFilterGain/1 -> Integrator/1
  Switch/1 -> Sum4/1
  h/1 -> Mux/1
  xl/1 -> Sum/2
  Sum1/1 -> Sum/1  "x (front bumber)"
  vf/1 -> Multiply/1
  Sum3/1 -> Sum2/2  "desired  gap"
  xf/1 -> Sum1/2
  Sum/1 -> Sum2/1, "gap "/1  "gap"
  Multiply/1 -> Sum3/1
  vLen/1 -> Sum1/1

== system gap_generation_single_veh/Lo/Longitudinal Adjustments for Lane Change/Veh Following ==
  eh : Inport
  ev : Inport  Port=2
  realInput : Inport  Port=3
  Anti-windup gain : Gain  Gain=sqrt(Ki/Kd)
  Integrator : Integrator
  Kd : Gain  Gain=Kd
  Ki : Gain  Gain=Ki
  Kp : Gain  Gain=Kp
  Saturation1 : Saturate  UpperLimit=maxHeadwayError  LowerLimit=minHeadwayError
  Scope : Scope  NumInputPorts=3
  Sum : Sum  Inputs=|-+
  Sum1 : Sum  Inputs=+++
  Sum5 : Sum  Inputs=-+|
  u : Outport
  wires:
  Sum/1 -> Anti-windup gain/1
  realInput/1 -> Sum/1
  Sum1/1 -> u/1, Sum/2
  eh/1 -> Saturation1/1
  Saturation1/1 -> Ki/1, Kp/1
  Kd/1 -> Sum1/3, Scope/3
  Kp/1 -> Sum1/2, Scope/2
  Integrator/1 -> Sum1/1, Scope/1
  Sum5/1 -> Integrator/1
  Anti-windup gain/1 -> Sum5/1
  Ki/1 -> Sum5/2
  ev/1 -> Kd/1

== system gap_generation_single_veh/Lo/Longitudinal Adjustments for Lane Change/Velocity Control ==
  note: Velocity control
  intReset : Inport
  ev : Inport  Port=2
  Integrator2 : Integrator  ExternalReset=rising
  Sum3 : Sum
  velKi : Gain  Gain=velKi
  velKp : Gain  Gain=velKp
  Out1 : Outport
  wires:
  intReset/1 -> Integrator2/2
  ev/1 -> Integrator2/1, velKp/1
  velKp/1 -> Sum3/1
  Sum3/1 -> Out1/1
  velKi/1 -> Sum3/2
  Integrator2/1 -> velKi/1

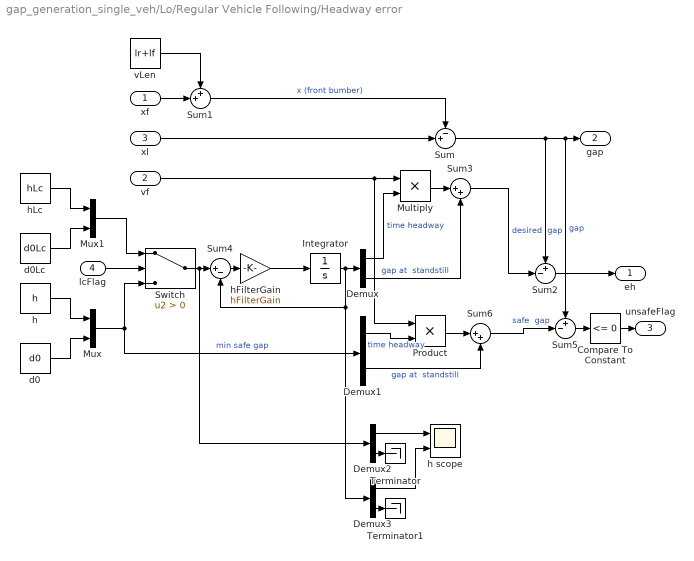
== system gap_generation_single_veh/Lo/Regular Vehicle Following/Headway error ==
  xf : Inport
  vf : Inport  Port=2
  xl : Inport  Port=3
  lcFlag : Inport  Port=4
  Compare To Constant : simulink/Logic and Bit Operations/Compare To Constant  relop=<=  const=0  OutDataTypeStr=boolean
  Demux{,1..3} (4 alike) : Demux  Outputs=2
  Integrator : Integrator  InitialCondition=[h d0]
  Multiply : Product
  Mux : Mux  Inputs=2
  Mux1 : Mux  Inputs=2
  Product : Product
  Sum : Sum  Inputs=-+|
  Sum1 : Sum  Inputs=++|
  Sum2 : Sum  Inputs=+-|
  Sum3 : Sum  Inputs=|++
  Sum4 : Sum  Inputs=|+-
  Sum5 : Sum  Inputs=+-|
  Sum6 : Sum  Inputs=|++
  Switch : Switch  Criteria=u2 > Threshold
  Terminator : Terminator
  Terminator1 : Terminator
  d0 : Constant  Value=d0
  d0Lc : Constant  Value=d0Lc
  h : Constant  Value=h
  h scope : Scope  NumInputPorts=2
  hFilterGain : Gain  Gain=hFilterGain
  hLc : Constant  Value=hLc
  vLen : Constant  Value=lr+lf
  eh : Outport
  "gap " : Outport  Port=2
  unsafeFlag : Outport  Port=3
  wires:
  Demux3/2 -> Terminator1/1
  Demux2/2 -> Terminator/1
  Demux3/1 -> h scope/2
  Demux2/1 -> h scope/1
  Sum6/1 -> Sum5/2  "safe  gap"
  Demux1/2 -> Sum6/2  "gap at  standstill"
  Product/1 -> Sum6/1
  Demux1/1 -> Product/2  "time headway"
  Compare To Constant/1 -> unsafeFlag/1
  Sum5/1 -> Compare To Constant/1
  hFilterGain/1 -> Integrator/1
  Demux/2 -> Sum3/2  "gap at  standstill"
  Demux/1 -> Multiply/2  "time headway"
  Mux1/1 -> Switch/1
  d0Lc/1 -> Mux1/2
  hLc/1 -> Mux1/1
  Mux/1 -> Switch/3, Demux1/1  "min safe gap"
  d0/1 -> Mux/2
  Sum2/1 -> eh/1
  lcFlag/1 -> Switch/2
  Integrator/1 -> Demux/1, Sum4/2, Demux3/1
  Sum4/1 -> hFilterGain/1
  Switch/1 -> Sum4/1, Demux2/1
  h/1 -> Mux/1
  xl/1 -> Sum/2
  Sum1/1 -> Sum/1  "x (front bumber)"
  vf/1 -> Multiply/1, Product/1
  Sum3/1 -> Sum2/2  "desired  gap"
  xf/1 -> Sum1/2
  Sum/1 -> Sum2/1, "gap "/1, Sum5/1  "gap"
  Multiply/1 -> Sum3/1
  vLen/1 -> Sum1/1

== system gap_generation_single_veh/Lo/Regular Vehicle Following/Veh Following ==
  eh : Inport
  ev : Inport  Port=2
  realInput : Inport  Port=3
  Enable : EnablePort
  Anti-windup gain : Gain  Gain=sqrt(Ki/Kd)
  Integrator : Integrator
  Kd : Gain  Gain=Kd
  Ki : Gain  Gain=Ki
  Kp : Gain  Gain=Kp
  Saturation1 : Saturate  UpperLimit=maxHeadwayError  LowerLimit=minHeadwayError
  Scope : Scope  NumInputPorts=3
  Sum : Sum  Inputs=|-+
  Sum1 : Sum  Inputs=+++
  Sum5 : Sum  Inputs=-+|
  u : Outport
  wires:
  Sum/1 -> Anti-windup gain/1
  realInput/1 -> Sum/1
  Sum1/1 -> u/1, Sum/2
  eh/1 -> Saturation1/1
  Saturation1/1 -> Ki/1, Kp/1
  Kd/1 -> Sum1/3, Scope/3
  Kp/1 -> Sum1/2, Scope/2
  Integrator/1 -> Sum1/1, Scope/1
  Sum5/1 -> Integrator/1
  Anti-windup gain/1 -> Sum5/1
  Ki/1 -> Sum5/2
  ev/1 -> Kd/1

== system gap_generation_single_veh/Lo/Regular Vehicle Following/Velocity Control ==
  note: Velocity control
  ev : Inport
  Enable : EnablePort
  Integrator2 : Integrator
  Sum3 : Sum
  velKi : Gain  Gain=velKi
  velKp : Gain  Gain=velKp
  Out1 : Outport
  wires:
  ev/1 -> Integrator2/1, velKp/1
  velKp/1 -> Sum3/1
  Sum3/1 -> Out1/1
  velKi/1 -> Sum3/2
  Integrator2/1 -> velKi/1

== system gap_generation_single_veh/p1/Longitudinal Adjustments for Lane Change/Headway error ==
  xf : Inport
  vf : Inport  Port=2
  xl : Inport  Port=3
  lcFlag : Inport  Port=4
  Demux : Demux  Outputs=2
  Integrator : Integrator  InitialCondition=h
  Multiply : Product
  Mux : Mux  Inputs=2
  Mux1 : Mux  Inputs=2
  Sum : Sum  Inputs=-+|
  Sum1 : Sum  Inputs=++|
  Sum2 : Sum  Inputs=+-|
  Sum3 : Sum  Inputs=|++
  Sum4 : Sum  Inputs=|+-
  Switch : Switch  Criteria=u2 > Threshold
  d0 : Constant  Value=d0
  d0Lc : Constant  Value=d0Lc
  h : Constant  Value=h
  hFilterGain : Gain  Gain=hFilterGain
  hLc : Constant  Value=hLc
  vLen : Constant  Value=lr+lf
  eh : Outport
  "gap " : Outport  Port=2
  wires:
  Demux/2 -> Sum3/2  "gap at  standstill"
  Demux/1 -> Multiply/2  "time headway"
  Mux1/1 -> Switch/1
  d0Lc/1 -> Mux1/2
  hLc/1 -> Mux1/1
  Mux/1 -> Switch/3
  d0/1 -> Mux/2
  Sum2/1 -> eh/1
  lcFlag/1 -> Switch/2
  Integrator/1 -> Demux/1, Sum4/2
  Sum4/1 -> hFilterGain/1
  hFilterGain/1 -> Integrator/1
  Switch/1 -> Sum4/1
  h/1 -> Mux/1
  xl/1 -> Sum/2
  Sum1/1 -> Sum/1  "x (front bumber)"
  vf/1 -> Multiply/1
  Sum3/1 -> Sum2/2  "desired  gap"
  xf/1 -> Sum1/2
  Sum/1 -> Sum2/1, "gap "/1  "gap"
  Multiply/1 -> Sum3/1
  vLen/1 -> Sum1/1

== system gap_generation_single_veh/p1/Longitudinal Adjustments for Lane Change/Veh Following ==
  eh : Inport
  ev : Inport  Port=2
  realInput : Inport  Port=3
  Anti-windup gain : Gain  Gain=sqrt(Ki/Kd)
  Integrator : Integrator
  Kd : Gain  Gain=Kd
  Ki : Gain  Gain=Ki
  Kp : Gain  Gain=Kp
  Saturation1 : Saturate  UpperLimit=maxHeadwayError  LowerLimit=minHeadwayError
  Scope : Scope  NumInputPorts=3
  Sum : Sum  Inputs=|-+
  Sum1 : Sum  Inputs=+++
  Sum5 : Sum  Inputs=-+|
  u : Outport
  wires:
  Sum/1 -> Anti-windup gain/1
  realInput/1 -> Sum/1
  Sum1/1 -> u/1, Sum/2
  eh/1 -> Saturation1/1
  Saturation1/1 -> Ki/1, Kp/1
  Kd/1 -> Sum1/3, Scope/3
  Kp/1 -> Sum1/2, Scope/2
  Integrator/1 -> Sum1/1, Scope/1
  Sum5/1 -> Integrator/1
  Anti-windup gain/1 -> Sum5/1
  Ki/1 -> Sum5/2
  ev/1 -> Kd/1

== system gap_generation_single_veh/p1/Longitudinal Adjustments for Lane Change/Velocity Control ==
  note: Velocity control
  intReset : Inport
  ev : Inport  Port=2
  Integrator2 : Integrator  ExternalReset=rising
  Sum3 : Sum
  velKi : Gain  Gain=velKi
  velKp : Gain  Gain=velKp
  Out1 : Outport
  wires:
  intReset/1 -> Integrator2/2
  ev/1 -> Integrator2/1, velKp/1
  velKp/1 -> Sum3/1
  Sum3/1 -> Out1/1
  velKi/1 -> Sum3/2
  Integrator2/1 -> velKi/1

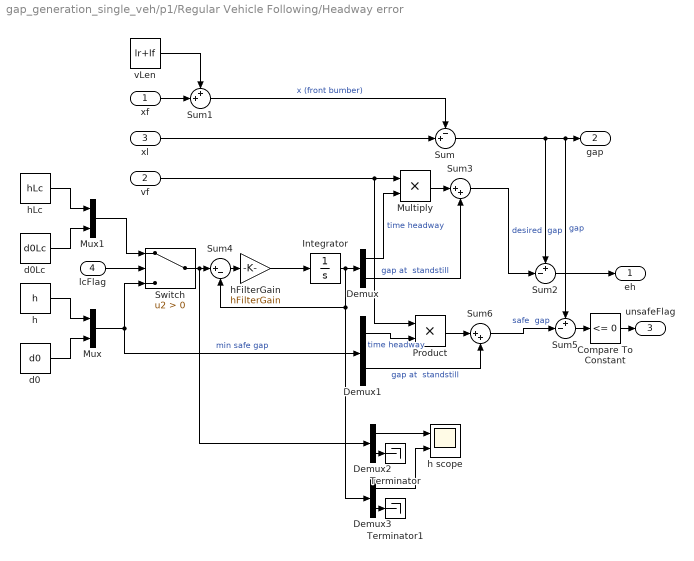
== system gap_generation_single_veh/p1/Regular Vehicle Following/Headway error ==
  xf : Inport
  vf : Inport  Port=2
  xl : Inport  Port=3
  lcFlag : Inport  Port=4
  Compare To Constant : simulink/Logic and Bit Operations/Compare To Constant  relop=<=  const=0  OutDataTypeStr=boolean
  Demux{,1..3} (4 alike) : Demux  Outputs=2
  Integrator : Integrator  InitialCondition=[h d0]
  Multiply : Product
  Mux : Mux  Inputs=2
  Mux1 : Mux  Inputs=2
  Product : Product
  Sum : Sum  Inputs=-+|
  Sum1 : Sum  Inputs=++|
  Sum2 : Sum  Inputs=+-|
  Sum3 : Sum  Inputs=|++
  Sum4 : Sum  Inputs=|+-
  Sum5 : Sum  Inputs=+-|
  Sum6 : Sum  Inputs=|++
  Switch : Switch  Criteria=u2 > Threshold
  Terminator : Terminator
  Terminator1 : Terminator
  d0 : Constant  Value=d0
  d0Lc : Constant  Value=d0Lc
  h : Constant  Value=h
  h scope : Scope  NumInputPorts=2
  hFilterGain : Gain  Gain=hFilterGain
  hLc : Constant  Value=hLc
  vLen : Constant  Value=lr+lf
  eh : Outport
  "gap " : Outport  Port=2
  unsafeFlag : Outport  Port=3
  wires:
  Demux3/2 -> Terminator1/1
  Demux2/2 -> Terminator/1
  Demux3/1 -> h scope/2
  Demux2/1 -> h scope/1
  Sum6/1 -> Sum5/2  "safe  gap"
  Demux1/2 -> Sum6/2  "gap at  standstill"
  Product/1 -> Sum6/1
  Demux1/1 -> Product/2  "time headway"
  Compare To Constant/1 -> unsafeFlag/1
  Sum5/1 -> Compare To Constant/1
  hFilterGain/1 -> Integrator/1
  Demux/2 -> Sum3/2  "gap at  standstill"
  Demux/1 -> Multiply/2  "time headway"
  Mux1/1 -> Switch/1
  d0Lc/1 -> Mux1/2
  hLc/1 -> Mux1/1
  Mux/1 -> Switch/3, Demux1/1  "min safe gap"
  d0/1 -> Mux/2
  Sum2/1 -> eh/1
  lcFlag/1 -> Switch/2
  Integrator/1 -> Demux/1, Sum4/2, Demux3/1
  Sum4/1 -> hFilterGain/1
  Switch/1 -> Sum4/1, Demux2/1
  h/1 -> Mux/1
  xl/1 -> Sum/2
  Sum1/1 -> Sum/1  "x (front bumber)"
  vf/1 -> Multiply/1, Product/1
  Sum3/1 -> Sum2/2  "desired  gap"
  xf/1 -> Sum1/2
  Sum/1 -> Sum2/1, "gap "/1, Sum5/1  "gap"
  Multiply/1 -> Sum3/1
  vLen/1 -> Sum1/1

== system gap_generation_single_veh/p1/Regular Vehicle Following/Veh Following ==
  eh : Inport
  ev : Inport  Port=2
  realInput : Inport  Port=3
  Enable : EnablePort
  Anti-windup gain : Gain  Gain=sqrt(Ki/Kd)
  Integrator : Integrator
  Kd : Gain  Gain=Kd
  Ki : Gain  Gain=Ki
  Kp : Gain  Gain=Kp
  Saturation1 : Saturate  UpperLimit=maxHeadwayError  LowerLimit=minHeadwayError
  Scope : Scope  NumInputPorts=3
  Sum : Sum  Inputs=|-+
  Sum1 : Sum  Inputs=+++
  Sum5 : Sum  Inputs=-+|
  u : Outport
  wires:
  Sum/1 -> Anti-windup gain/1
  realInput/1 -> Sum/1
  Sum1/1 -> u/1, Sum/2
  eh/1 -> Saturation1/1
  Saturation1/1 -> Ki/1, Kp/1
  Kd/1 -> Sum1/3, Scope/3
  Kp/1 -> Sum1/2, Scope/2
  Integrator/1 -> Sum1/1, Scope/1
  Sum5/1 -> Integrator/1
  Anti-windup gain/1 -> Sum5/1
  Ki/1 -> Sum5/2
  ev/1 -> Kd/1

== system gap_generation_single_veh/p1/Regular Vehicle Following/Velocity Control ==
  note: Velocity control
  ev : Inport
  Enable : EnablePort
  Integrator2 : Integrator
  Sum3 : Sum
  velKi : Gain  Gain=velKi
  velKp : Gain  Gain=velKp
  Out1 : Outport
  wires:
  ev/1 -> Integrator2/1, velKp/1
  velKp/1 -> Sum3/1
  Sum3/1 -> Out1/1
  velKi/1 -> Sum3/2
  Integrator2/1 -> velKi/1

== stateflow chart gap_generation_single_veh/Lo/Chart ==
  state RegVehFoll
    during:
    u = regVehFollU;
  state AdjForLaneChange
    during:
    u = min(regVehFollU, virtualVehFollU);
  (default) -> RegVehFoll
  RegVehFoll -> AdjForLaneChange : [startAdjustment==1]
  data: regVehFollU input size=1; virtualVehFollU input size=1; startAdjustment input size=1; u output size=1
